simulink model "complimentary_filter"  (R2017b)
settings: Solver=FixedStepDiscrete  StartTime=0.0  StopTime=inf  RelTol=1e-3  EnableMultiTasking=on
undefined symbols (not defined in the file): DiscIntNeverNeededParam
libraries: beaglebonebluelib x2, simulink_extras x1
settings Model: FPTRunName=Active  SimulationMode=external  ExtModeTrigDuration=2  Creator=The MathWorks, Inc.  LastModifiedBy=pthb3
settings SolverCC: PositivePriorityOrder=on
settings DataIOCC: LimitDataPoints=on  SaveFormat=Array
settings OptimizationCC: ExpressionDepthLimit=2147483647  LifeSpan=Inf  MaxStackSize=64
settings DebuggingCC: UnderspecifiedInitializationDetection=Classic  MergeDetectMultiDrivingBlocksExec=none  FcnCallInpInsideContextMsg=warning  AllowSymbolicDim=off  StateNameClashWarn=warning  SFUnexpectedBacktrackingDiag=warning  SFNoUnconditionalDefaultTransitionDiag=warning  SFExecutionAtInitializationDiag=none
settings HardwareCC: ProdBitPerPointer=32  ProdBitPerSizeT=32  ProdBitPerPtrDiffT=32  ProdLargestAtomicInteger=Long  ProdLargestAtomicFloat=Double  ProdWordSize=32  ProdHWDeviceType=ARM Compatible->ARM Cortex  UseEmbeddedCoderFeatures=off
settings ModelReferenceCC: PropagateSignalLabelsOutOfModel=off
settings RTWCC: SystemTargetFile=ert.tlc  HardwareBoard=BeagleBone Blue  TemplateMakefile=ert_default_tmf  RTWVerbose=off  Toolchain=GNU GCC BeagleBone Blue
settings CodeAppCC: StateflowObjectComments=on
settings ERTTargetCC: MultiwordLength=2048  ERTCustomFileBanners=off  SupportContinuousTime=on  SupportNonInlinedSFcns=on  RemoveResetFunc=off  SupportVariableSizeSignals=on  ModelStepFunctionPrototypeControlCompliant=off  ConvertIfToSwitch=off  SuppressUnreachableDefaultCases=off
settings ConfigComp: CovMetricSettings=dw  CovHtmlReporting=on  CovSaveCumulativeToWorkspaceVar=on  CovSaveSingleToWorkspaceVar=on  CovExternalEMLEnable=off  CovSFcnEnable=off

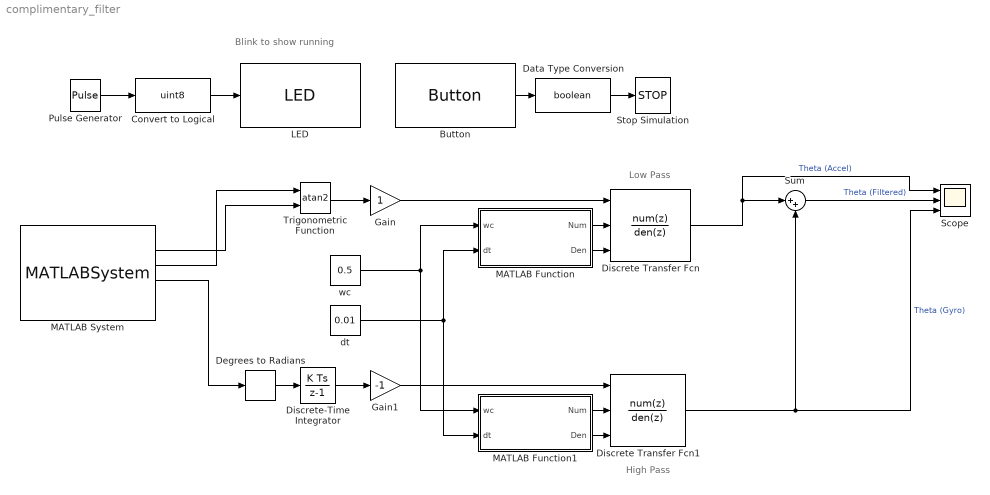
== system complimentary_filter ==
  note: Blink to show running
  note: Low Pass
  note: High Pass
  Button : beaglebonebluelib/Button  Button=Mode  SampleTime=0.1  SimulateUsing=Code generation
      settings: SourceProductName=Simulink Coder Support Package for BeagleBone Blue Hardware
  Convert to Logical : DataTypeConversion  OutDataTypeStr=uint8
  Data Type Conversion : DataTypeConversion  OutDataTypeStr=boolean
  Degrees to Radians : simulink_extras/Transformations/Degrees to Radians
  Discrete Transfer Fcn : DiscreteTransferFcn  NumeratorSource=Input port  DenominatorSource=Input port  Denominator=[1]  a0EqualsOne=on
      settings: InputPortMap=u0,p1,p3
  Discrete Transfer Fcn1 : DiscreteTransferFcn  NumeratorSource=Input port  DenominatorSource=Input port  Denominator=[1]  a0EqualsOne=on
      settings: InputPortMap=u0,p1,p3
  Discrete-Time Integrator : DiscreteIntegrator  InitialConditionSetting=State (most efficient)  SampleTime=-1  ICPrevOutput=DiscIntNeverNeededParam  ICPrevScaledInput=DiscIntNeverNeededParam
  Gain : Gain
  Gain1 : Gain  Gain=-1
  LED : beaglebonebluelib/LED  LED=Green
      settings: SourceProductName=Simulink Coder Support Package for BeagleBone Blue Hardware
  MATLAB Function : MATLAB Function  TreatAsAtomicUnit=on
  MATLAB Function1 : MATLAB Function  TreatAsAtomicUnit=on
  MATLAB System : MATLABSystem  System=beagleboneblue.fccr_bbblueIMU  SampleTime=0.01
      mask Type: beagleboneblue.fccr_bbblueIMU
      mask Display:
      | color('white');
      | plot([100,100,100,100]*1,[100,100,100,100]*1);
      | plot([100,100,100,100]*0,[100,100,100,100]*0);
      | color('blue');
      | text(100, 92, ' BB BLUE ', 'horizontalAlignment', 'right');
      | color('black');
      | text(52,52,' IMU','horizontalAlignment','center');
      | color('black');
  Pulse Generator : DiscretePulseGenerator  Period=10  PulseWidth=5  SampleTime=0.1
  Scope : Scope  NumInputPorts=3
  Stop Simulation : Stop
  Sum : Sum  Inputs=|++
  Trigonometric Function : Trigonometry  Operator=atan2
  dt : Constant  Value=0.01
  wc : Constant  Value=0.5
  wires:
  Convert to Logical/1 -> LED/1
  Pulse Generator/1 -> Convert to Logical/1
  dt/1 -> MATLAB Function1/2(dt), MATLAB Function/2(dt)
  Gain/1 -> Discrete Transfer Fcn/1
  MATLAB Function1/2(Den) -> Discrete Transfer Fcn1/3
  wc/1 -> MATLAB Function1/1(wc), MATLAB Function/1(wc)
  MATLAB Function/2(Den) -> Discrete Transfer Fcn/3
  MATLAB System/3 -> Trigonometric Function/1
  MATLAB Function1/1(Num) -> Discrete Transfer Fcn1/2
  Sum/1 -> Scope/2  "Theta (Filtered)"
  Discrete Transfer Fcn/1 -> Scope/1, Sum/1  "Theta (Accel)"
  MATLAB System/4 -> Degrees to Radians/1
  MATLAB Function/1(Num) -> Discrete Transfer Fcn/2
  Discrete-Time Integrator/1 -> Gain1/1
  Trigonometric Function/1 -> Gain/1
  Discrete Transfer Fcn1/1 -> Sum/2, Scope/3  "Theta (Gyro)"
  MATLAB System/2 -> Trigonometric Function/2
  Degrees to Radians/1 -> Discrete-Time Integrator/1
  Gain1/1 -> Discrete Transfer Fcn1/1
  Button/1 -> Data Type Conversion/1
  Data Type Conversion/1 -> Stop Simulation/1

== matlab function complimentary_filter/MATLAB Function1 ==
  data: wc input; Num output; dt input; Den output
function [Num, Den] = first_order_hp(wc,dt)
%#codegen
Num = [1 -1];
Den = [1 (wc*dt - 1)];

== matlab function complimentary_filter/MATLAB Function ==
  data: wc input; Num output; dt input; Den output
function [Num, Den] = first_order_lp(wc,dt)
%#codegen
Num = [0 wc*dt];
Den = [1 (wc*dt - 1)];
